simulink library "Lib_AP_Motors"  (R2014b)
settings: Solver=ode45  StartTime=0.0  StopTime=10.0  RelTol=1e-3
values from neighbouring files (symbols this model uses):
  DEG_TO_RAD = (M_PI/180.0)    (= 0.0174532925199)    [LoadParameters.m]
libraries: Lib_AP_Math x2
settings Model: Creator=Ehang  LastModifiedBy=Ehang

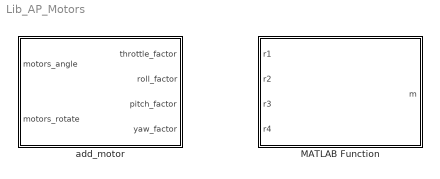
== system Lib_AP_Motors ==
  MATLAB Function : MATLAB Function  TreatAsAtomicUnit=on
  add_motor : Subsystem

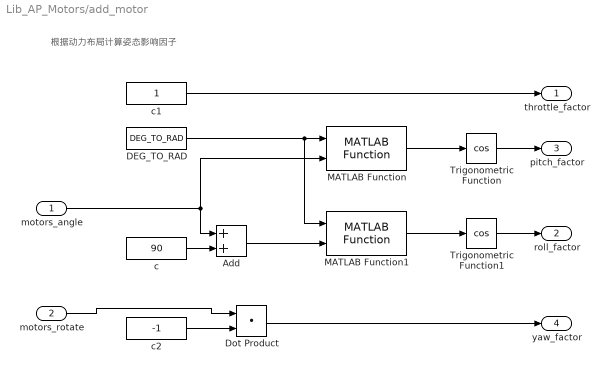
== system Lib_AP_Motors/add_motor ==
  note: 根据动力布局计算姿态影响因子
  motors_angle : Inport
  motors_rotate : Inport  Port=2
  Add : Sum
  DEG_TO_RAD : Constant  Description=低通滤波器的时间常数  Value=DEG_TO_RAD
  Dot Product : DotProduct  InputSameDT=on  OutDataTypeStr=Inherit: Inherit via internal rule
  MATLAB Function : Lib_AP_Math/MATLAB Function
  MATLAB Function1 : Lib_AP_Math/MATLAB Function
  Trigonometric Function : Trigonometry  Operator=cos
  Trigonometric Function1 : Trigonometry  Operator=cos
  c : Constant  Description=低通滤波器的时间常数  Value=90
  c1 : Constant  Description=低通滤波器的时间常数
  c2 : Constant  Description=低通滤波器的时间常数  Value=-1
  throttle_factor : Outport
  roll_factor : Outport  Port=2
  pitch_factor : Outport  Port=3
  yaw_factor : Outport  Port=4
  wires:
  DEG_TO_RAD/1 -> MATLAB Function1/1, MATLAB Function/1
  motors_rotate/1 -> Dot Product/1
  c/1 -> Add/2
  Dot Product/1 -> yaw_factor/1
  Add/1 -> MATLAB Function1/2
  c2/1 -> Dot Product/2
  Trigonometric Function1/1 -> roll_factor/1
  c1/1 -> throttle_factor/1
  MATLAB Function/1 -> Trigonometric Function/1
  Trigonometric Function/1 -> pitch_factor/1
  MATLAB Function1/1 -> Trigonometric Function1/1
  motors_angle/1 -> MATLAB Function/2, Add/1

== matlab function Lib_AP_Motors/MATLAB Function ==
  data: r1 input size=[1,4]; r2 input size=[1,4]; m output; r3 input size=[1,4]; r4 input size=[1,4]
function m= r_to_m(r1,r2,r3,r4)
m=[r1;r2;r3;r4];
